simulink model "P10"  (R2022b)
settings: Solver=VariableStepAuto  StartTime=0.0  StopTime=10.0  RelTol=1e-3
settings Model: Creator=Khaled  LastModifiedBy=Khaled

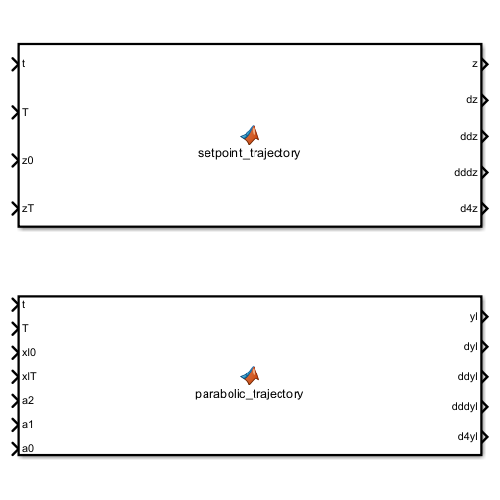
[thumbnail: Simulink's stored preview of the top-level diagram]
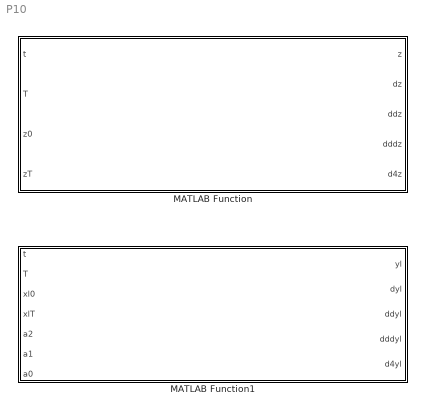
== system P10 ==
  MATLAB Function : MATLAB Function  TreatAsAtomicUnit=on
  MATLAB Function1 : MATLAB Function  TreatAsAtomicUnit=on

== matlab function P10/MATLAB Function1 ==
  data: t input; yl output; T input; xl0 input; xlT input; a2 input; a1 input; a0 input; dyl output; ddyl output; dddyl output; d4yl output
function [yl, dyl, ddyl, dddyl, d4yl] = parabolic_trajectory(t, T, xl0, xlT, a2, a1, a0)
    % Polynomial Coefficients for xl
    p5 = 126; p6 = -420; p7 = 540; p8 = -315; p9 = 70;
    tau = t / T; % Normalized time

    % Polynomial Trajectory for xl
    xl = xl0 + (xlT - xl0) * (p5 * tau^5 + p6 * tau^6 + p7 * tau^7 + p8 * tau^8 + p9 * tau^9);
    dxl = (xlT - xl0) / T * (5 * p5 * tau^4 + 6 * p6 * tau^5 + 7 * p7 * tau^6 + 8 * p8 * tau^7 + 9 * p9 * tau^8);
    ddxl = (xlT - xl0) / T^2 * (20 * p5 * tau^3 + 30 * p6 * tau^4 + 42 * p7 * tau^5 + 56 * p8 * tau^6 + 72 * p9 * tau^7);

    % Parabolic Trajectory
    yl = a2 * xl^2 + a1 * xl + a0;
    dyl = 2 * a2 * xl * dxl + a1 * dxl;
    ddyl = 2 * a2 * (dxl^2 + xl * ddxl);
    dddyl = 2 * a2 * (2 * dxl * ddxl + xl * 0); % Use appropriate higher derivatives
    d4yl = 2 * a2 * (3 * ddxl^2); % Compute higher derivatives if needed
end

== matlab function P10/MATLAB Function ==
  data: t input; z output; T input; z0 input; zT input; dz output; ddz output; dddz output; d4z output
function [z, dz, ddz, dddz, d4z] = setpoint_trajectory(t, T, z0, zT)
    % Polynomial Coefficients
    p5 = 126; p6 = -420; p7 = 540; p8 = -315; p9 = 70;
    tau = t / T; % Normalized time

    % Polynomial Trajectory
    z = z0 + (zT - z0) * (p5 * tau^5 + p6 * tau^6 + p7 * tau^7 + p8 * tau^8 + p9 * tau^9);

    % Derivatives
    dz = (zT - z0) / T * (5 * p5 * tau^4 + 6 * p6 * tau^5 + 7 * p7 * tau^6 + 8 * p8 * tau^7 + 9 * p9 * tau^8);
    ddz = (zT - z0) / T^2 * (20 * p5 * tau^3 + 30 * p6 * tau^4 + 42 * p7 * tau^5 + 56 * p8 * tau^6 + 72 * p9 * tau^7);
    dddz = (zT - z0) / T^3 * (60 * p5 * tau^2 + 120 * p6 * tau^3 + 210 * p7 * tau^4 + 336 * p8 * tau^5 + 504 * p9 * tau^6);
    d4z = (zT - z0) / T^4 * (120 * p5 * tau + 360 * p6 * tau^2 + 840 * p7 * tau^3 + 1680 * p8 * tau^4 + 3024 * p9 * tau^5);
end
